simulink model "tqdtqr_rebuild_V3"  (R2021b)
settings: Solver=VariableStepAuto  StartTime=0.0  StopTime=10.0  RelTol=1e-3
undefined symbols (not defined in the file): ATQD_AfterTqMinGain_X_Deg, ATQD_APSCreepBaseTqD_X_kph, ATQD_APSCreepBaseTqD_Y_Deg, ATQD_APSCreepBaseTqR_X_kph, ATQD_APSCreepBaseTqR_Y_Deg, ATQD_APSCreepIterm_X_kph, ATQD_APSCreepIterm_Y_kph, ATQD_APSCreepPterm_X_kph, ATQD_APSCreepPterm_Y_kph, ATQD_APSDecReq_X_kph, ATQD_APSDecReq_Y_mps2, ATQD_APSDecReqCMD_X_kph, ATQD_APSDecReqTs_X_pct, ATQD_APSDecTimeGain_X_Deg, ATQD_APSDecTimeGain_Y_s, ATQD_APSReqLowSpd_X_Deg, ATQD_AutoHoldReleaseBPS_X_Deg, ATQD_AWDLoadTrqnsGain_X_kg, ATQD_AWDLoadTrqnsGain_Y_pct, ATQD_BOSEnBPSPosn_X_kph, ATQD_BOSMap_X_rpm, ATQD_BOSMap_Y_pct, ATQD_CreepBaseTqD_X_kph, ATQD_CreepBaseTqD_Y_Deg, ATQD_CreepBaseTqR_X_kph, ATQD_CreepBaseTqR_Y_Deg, ATQD_CreepBPSDisPosn_X_Deg, ATQD_CreepBPSDisPosnR_X_Deg, ATQD_CreepBPSEnPosn_X_Deg, ATQD_CreepBPSEnPosnR_X_Deg, ATQD_CreepDeltaTq_X_kph, ATQD_CreepIterm_X_kph, ATQD_CreepIterm_Y_kph, ATQD_CreepItermMaxLimit_X_pct, ATQD_CreepPreloadTime_X_kph, ATQD_CreepPreloadTq_X_kph, ATQD_CreepPreloadTq_Y_s, ATQD_CreepProtTq_X_Deg, ATQD_CreepPterm_X_kph, ATQD_CreepPterm_Y_kph, ATQD_CreepRrTqSpRat_X_rpm, ATQD_CreepRrTqSpRat_Y_Nm, ATQD_CreepTargetSpdD_X_pct, ATQD_CreepTargetSpdR_X_pct, ATQD_CreepUpLimitTq_X_rpm, ATQD_DecIneOPDHoldEnDelay_X_Deg, ATQD_DecIneOPDHoldEnDelay_Y_bar, ATQD_ECOTqMapD_X_rpm, ATQD_ECOTqMapD_Y_pct, ATQD_EMTqMapD_X_rpm, ATQD_EMTqMapD_Y_pct, ATQD_EOPDTqMapDCon_X_rpm, ATQD_EOPDTqMapDCon_Y_Deg, ATQD_EstInitVehWeight_X_c, ATQD_FAfterTqCMDGain_X_rpm, ATQD_FAfterTqCMDGain_Y_pct, ATQD_ForceLowSpd_X_Deg, ATQD_ForcePLimitSpd_X_Deg, ATQD_FrLossMAPLowV_X_rpm, ATQD_FrLossMAPLowV_Y_Nm ... (+949)
libraries: simulink x235, hcu_lib x208, tqr x63, tqd x6
(part 16 of 37)

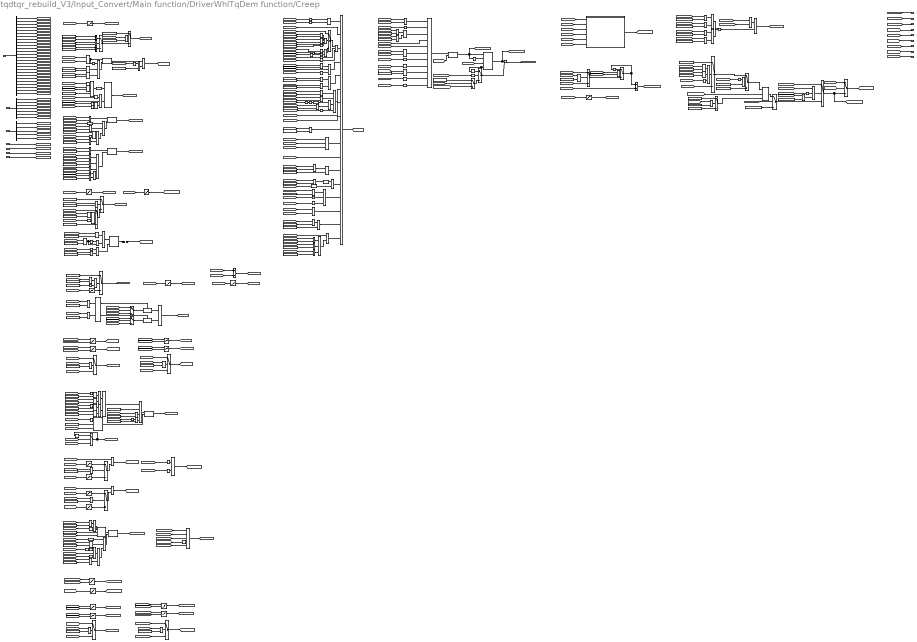
== system tqdtqr_rebuild_V3/Input_Convert/Main function/DriverWhlTqDem function/Creep ==
  note: Calculate creep torque with offset
  note: Creep control reset offset torque
  note: Creep Tq determination
  note: Creep enable parameters
  note: Creep disable parameters
  note: Output final creep torque
  note: Protection condition
  note: Determine brake pedal depth
  note: PI control get torque offset
  note: Preload torque / protect torque
  note: Calculate I value with vehicle speed and error speed
  note: Calculate P value with vehicle speed and error speed
  note: Calculate torque shift R with road slope
  note: Caluclate torque in shift D with road slope
  note: Get error speed from creep speed and vehicle speed
  note: Detemine slope degree
  note: Creep disable judgement
  note: Wheel Status Disable Creep Judgment
  note: Creep enable judgement
  note: calculate creep final speed
  note: Parameters
  note: Creep disable and enable
  note: Creep Tq calculation
  note: Creep offset Tq calculation
  BSCPIn_outputs : Inport
  BSignalConvert_outputs : Inport  Port=2
  BFunction_outputs : Inport  Port=3
  VTQD_PedalMapWhlTq_Nm : Inport  Port=4
  VTQD_LoSpdBrkCtrl_flg : Inport  Port=5
  VTQD_PreLoadPreEn_flg : Inport  Port=6
  VTQD_PedAccTqEn_flg : Inport  Port=7
  AND{,4..7,11..12,15,17,19..26,29} (18 alike) : Logic  AllPortsSameDT=off  OutDataTypeStr=boolean
  AND{1..3,8,13..14,18} (7 alike) : Logic  Inputs=3  AllPortsSameDT=off  OutDataTypeStr=boolean
  AND16 : Logic  Operator=OR  Inputs=3  AllPortsSameDT=off  OutDataTypeStr=boolean
  AND27 : Logic  Inputs=4  AllPortsSameDT=off  OutDataTypeStr=boolean
  Abs : Abs
  Add : Sum  Inputs=+-
  Add1 : Sum
  Add2 : Sum
  Add4 : Sum
  Bus Selector : BusSelector  OutputSignals=VTQD_LowIdleAccPedal_flg,VINP_VehSpeed_kph,VINP_AVHActive_flg,VTQD_ActBPSPosn_pct,VINP_RrRBCActive_flg,VINP_FrEDURealTMTq_Nm,VINP_RrEDURealTMTq_Nm,VINP_FrRBCActive_flg,VVMC_ADASActive_flg,task_time_s,VVMC_APSSpeedCMD_kph,VVMC_APSActive_flg,VVMC_APSReq_enum,VVMC_EstSlope_Deg,VPMM_PowerSta_enum,VINP_EPBSta_enum,VTQD_ActAPSPosn_pct,VVMC_CAASActive_flg,VINP_FrPTCSActive_flg,VINP_RrPTCSActive_flg,VDDM_EPB1Err_flg,VDDM_ESC5Err_flg,VDDM_EPBSigErrCFS_flg,VDDM_VehMalfunLevel_enum,VTQD_LimpHomeAct_flg,VDDM_VCURAPSErrLv2_flg
  Bus Selector1 : BusSelector  OutputSignals=VTQD_RegenMode_enum,VTQD_TMRotateDirction_enum,VTQD_RDCActive_enum,VTQD_BrkSwSta_flg,VTQD_VehActSpd_kph,VTQD_TqTargetShaftSpd_rpm,VTQD_CreepON_flg
  Bus Selector2 : BusSelector  OutputSignals=VTQD_GearActualPosn_enum,VTQD_ActWhlSkipSta_enum,VTQD_APSReq_enum,VTQD_APSReqTimer_s,VTQD_OPDHoldEnRel_flg
  Constant1 : Constant  Value=KTQD_APSCMDEnCreepSpd_kph
  Constant{10..12,21,25,58,62,82} (8 alike) : Constant  Value=ENUM_GEARACTUALPOSN_D
  Constant13 : Constant  Value=KTQD_CreepEnableSpd_kph
  Constant14 : Constant  Value=KTQD_APSCreepLowLimitTq_Nm
  Constant15 : Constant  Value=ZERO_FLOAT
  Constant17 : Constant  Value=ENUM_RDCACTSTA_NOREQUEST
  Constant18 : Constant  Value=ENUM_APSREQ_DECELCTRL  OutDataTypeStr=uint8
  Constant{2,9,20,35..36,38,42..44,49,81} (11 alike) : Constant  Value=ENUM_GEARACTUALPOSN_R
  Constant22 : Constant  Value=KTQD_CreepLowLimitTq_Nm
  Constant23 : Constant  Value=KTQD_CreepPrLoadEnSpd_kph
  Constant24 : Constant  Value=ENUM_RDCACTSTA_NOREQUEST
  Constant26 : Constant  Value=KTQD_CreepDisableSpdofst_kph
  Constant27 : Constant  Value=KTQD_CreepEnableSpdR_kph
  Constant28 : Constant  Value=KTQD_CreepDisableSpdofstR_kph
  Constant29 : Constant  Value=KTQD_CreepEnableSpdR_kph
  Constant{3,87..90} (5 alike) : Constant  Value=KTQD_APSCreepParOvrd_flg
  Constant37 : Constant  Value=ENUM_TMROTATEDIRECTACT_REVERSE  OutDataTypeStr=Inherit: Inherit via back propagation
  Constant39 : Constant  Value=ENUM_TMROTATEDIRECTACT_FORWARD  OutDataTypeStr=Inherit: Inherit via back propagation
  Constant{4,8,52,54,59,64} (6 alike) : Constant  Value=ENUM_REGENLEVEL_OPD
  Constant40 : Constant  Value=KTQD_RBCCreepRecTq_Nm
  Constant41 : Constant  Value=KTQD_RBCCreepRecTq_Nm
  Constant45 : Constant  Value=ENUM_POWERSTA_READY
  Constant46 : Constant  Value=KTQD_CreepEnableSpd_kph
  Constant5 : Constant  Value=ENUM_APSREQ_BRKHOLD  OutDataTypeStr=uint8
  Constant50 : Constant  Value=KTQD_OPDCreepTargetSpdD_kph
  Constant51 : Constant  Value=KTQD_APSReqDisCreep_flg  OutDataTypeStr=uint8
  Constant53 : Constant  Value=KTQD_APSReqDelayTime_s
  Constant55 : Constant  Value=ENUM_EPBSTA_APPLIED  OutDataTypeStr=uint8
  Constant56 : Constant  Value=KTQD_APSReqDisCreep_flg
  Constant6 : Constant  Value=ENUM_GEARACTUALPOSN_P
  Constant60 : Constant  Value=KTQD_OPDCreepDUpLimitTq_Nm
  Constant61 : Constant  Value=KTQD_CreepDisPedTqSpd_kph
  Constant63 : Constant  Value=KTQD_CreepAPSPosn2Launch_pct
  Constant65 : Constant  Value=ENUM_APSREQ_DECELCTRL  OutDataTypeStr=uint8
  Constant66 : Constant  Value=KTQD_TCSCreepDisSpdSW_flg
  Constant67 : Constant  Value=KTQD_TCSCreepDisSpd_kph
  Constant68 : Constant  Value=ENUM_SKIPDISCREEP_LOW
  Constant69 : Constant  Value=KTQD_LowSkipDisCreepDelay_s
  Constant7 : Constant  Value=ENUM_GEARACTUALPOSN_N
  Constant70 : Constant  Value=ENUM_EPBSTA_APPLIED
  Constant71 : Constant  Value=ENUM_SKIPDISCREEP_MEDIUM
  Constant72 : Constant  Value=ENUM_EPBSTA_APPLIED
  Constant73 : Constant  Value=ENUM_SKIPDISCREEP_NORMAL
  Constant74 : Constant  Value=ENUM_SKIPDISCREEP_NORMAL
  Constant75 : Constant  Value=ENUM_SKIPDISCREEP_HIGH
  Constant76 : Constant  Value=ENUM_GEARACTUALPOSN_N
  Constant77 : Constant  Value=ENUM_GEARACTUALPOSN_P
  Constant78 : Constant  Value=ENUM_EPBSTA_APPLIED
  Constant79 : Constant  Value=ENUM_SKIPDISCREEP_NORMAL
  Constant80 : Constant  Value=KTQD_RAPSCreepPreloadSetTime_s
  Constant83 : Constant  Value=KTQD_CreepSlopeLatchSW_flg
  Constant84 : Constant  Value=KTQD_CreepGradeLatchSpd_kph
  Constant85 : Constant  Value=KTQD_CreepLatchGradeDev_Deg
  Constant86 : Constant  Value=KTQD_CreepGradeRecTime_s
  Constant91 : Constant  Value=KTQD_TCSCreepSW_flg
  Constant93 : Constant  Value=KTQD_MALCreepUpLimitTq_Nm
  Constant94 : Constant  Value=ENUM_VEHMALFUNLEVEL_LEVEL3
  Constant97 : Constant  Value=KTQD_FailsafeActiveSW_flg
  Constant98 : Constant  Value=KTQD_FailsafeActiveSW_flg
  Constant99 : Constant  Value=KTQD_FailsafeActiveSW_flg
  Data Type Conversion : DataTypeConversion
  Delay : Delay  DelayLength=1
  Delay1 : Delay  DelayLength=1
  Delay10 : Delay  DelayLength=1  InitialCondition=single(0)
      settings: AttributesFormatString=%<InitialCondition>
  Delay{2..3,6..7} (4 alike) : Delay  DelayLength=1  InitialCondition=boolean(0)
      settings: AttributesFormatString=%<InitialCondition>
  Delay4 : Delay  DelayLength=1  InitialCondition=uint8 (0)
      settings: AttributesFormatString=%<InitialCondition>
  Delay5 : Delay  DelayLength=1  InitialCondition=uint8 (0)
      settings: AttributesFormatString=%<InitialCondition>
  Delay8 : Delay  DelayLength=1  InitialCondition=boolean (0)
      settings: AttributesFormatString=%<InitialCondition>
  Delay9 : Delay  DelayLength=1  InitialCondition=single (0)
      settings: AttributesFormatString=%<InitialCondition>
  DelayEnable : hcu_lib/Basic_Blocks/DelayEnable
  DelayEnable1 : hcu_lib/Basic_Blocks/DelayEnable
  Detect Change : simulink/Logic and Bit Operations/Detect Change  vinit=0  OutDataTypeStr=boolean
  Detect Change1 : simulink/Logic and Bit Operations/Detect Change  vinit=0  OutDataTypeStr=boolean
  Detect Change2 : simulink/Logic and Bit Operations/Detect Change  vinit=0  OutDataTypeStr=boolean
  Detect Increase : simulink/Logic and Bit Operations/Detect Increase  vinit=0  OutDataTypeStr=boolean
  Detect Increase1 : simulink/Logic and Bit Operations/Detect Increase  vinit=0.0  OutDataTypeStr=boolean
  Equal{4,6..8,10..16,19..31,33..54} (46 alike) : RelationalOperator  Operator===  OutDataTypeStr=boolean  RndMeth=Simplest
  Equal17 : RelationalOperator  Operator=<=  OutDataTypeStr=boolean  RndMeth=Simplest
  Equal18 : RelationalOperator  Operator=~=  OutDataTypeStr=boolean  RndMeth=Simplest
  Equal32 : RelationalOperator  OutDataTypeStr=boolean  RndMeth=Simplest
  Equal5 : RelationalOperator  Operator=<=  OutDataTypeStr=boolean  RndMeth=Simplest
  Equal55 : RelationalOperator  OutDataTypeStr=boolean  RndMeth=Simplest
  Equal9 : RelationalOperator  Operator=<=  OutDataTypeStr=boolean  RndMeth=Simplest
  GreaterThan : RelationalOperator  Operator=>  OutDataTypeStr=boolean  RndMeth=Simplest
  GreaterThan1 : RelationalOperator  Operator=>  OutDataTypeStr=boolean  RndMeth=Simplest
  GreaterThan2 : RelationalOperator  OutDataTypeStr=boolean  RndMeth=Simplest
  GreaterThan3 : RelationalOperator  Operator=>  OutDataTypeStr=boolean  RndMeth=Simplest
  GreaterThan4 : RelationalOperator  Operator=<=  OutDataTypeStr=boolean  RndMeth=Simplest
  Ground2 : Ground
  If : If  NumInputs=2  IfExpression=u1 ~= 0  ElseIfExpressions=u2 ~= 0  ShowElse=off
  If Action Subsystem : Subsystem  TreatAsAtomicUnit=on
  If Action Subsystem1 : Subsystem  TreatAsAtomicUnit=on
  Logical Operator{,8..11} (5 alike) : Logic  Operator=NOT  AllPortsSameDT=off  OutDataTypeStr=boolean
  Logical Operator{4,6,15..16,18} (5 alike) : Logic  AllPortsSameDT=off  OutDataTypeStr=boolean
  Logical Operator3 : Logic  Inputs=11  AllPortsSameDT=off  OutDataTypeStr=boolean
  Logical Operator5 : Logic  Operator=OR  AllPortsSameDT=off  OutDataTypeStr=boolean
  Logical Operator7 : Logic  Inputs=3  AllPortsSameDT=off  OutDataTypeStr=boolean
  MTQD_APSCreepBaseTqD_Z_Nm : Lookup_n-D  BreakpointsForDimension1=ATQD_APSCreepBaseTqD_Y_Deg  BreakpointsForDimension2=ATQD_APSCreepBaseTqD_X_kph  Table=MTQD_APSCreepBaseTqD_Z_Nm  ExtrapMethod=Clip  InternalRulePriority=Speed  RndMeth=Simplest  InputSameDT=on
      settings: InputPortMap=u0,u1
  MTQD_APSCreepBaseTqR_Z_Nm : Lookup_n-D  BreakpointsForDimension1=ATQD_APSCreepBaseTqR_Y_Deg  BreakpointsForDimension2=ATQD_APSCreepBaseTqR_X_kph  Table=MTQD_APSCreepBaseTqR_Z_Nm  ExtrapMethod=Clip  InternalRulePriority=Speed  RndMeth=Simplest  InputSameDT=on
      settings: InputPortMap=u0,u1
  MTQD_APSCreepIterm_Z_Nm : Lookup_n-D  BreakpointsForDimension1=ATQD_APSCreepIterm_Y_kph  BreakpointsForDimension2=ATQD_APSCreepIterm_X_kph  Table=MTQD_APSCreepIterm_Z_Nm  ExtrapMethod=Clip  InternalRulePriority=Speed  RndMeth=Simplest  InputSameDT=on
      settings: InputPortMap=u0,u1
  MTQD_APSCreepPterm_Z_Nm : Lookup_n-D  BreakpointsForDimension1=ATQD_APSCreepPterm_Y_kph  BreakpointsForDimension2=ATQD_APSCreepPterm_X_kph  Table=MTQD_APSCreepPterm_Z_Nm  ExtrapMethod=Clip  InternalRulePriority=Speed  RndMeth=Simplest  InputSameDT=on
      settings: InputPortMap=u0,u1
  MTQD_CreepBPSDisPosnR_Y_pct : Lookup_n-D  NumberOfTableDimensions=1  BreakpointsForDimension1=ATQD_CreepBPSDisPosnR_X_Deg  Table=MTQD_CreepBPSDisPosnR_Y_pct  ExtrapMethod=Clip  InternalRulePriority=Speed  RndMeth=Simplest  InputSameDT=on
  MTQD_CreepBPSDisPosn_Y_pct : Lookup_n-D  NumberOfTableDimensions=1  BreakpointsForDimension1=ATQD_CreepBPSDisPosn_X_Deg  Table=MTQD_CreepBPSDisPosn_Y_pct  ExtrapMethod=Clip  InternalRulePriority=Speed  RndMeth=Simplest  InputSameDT=on
  MTQD_CreepBPSEnPosnR_Y_pct : Lookup_n-D  NumberOfTableDimensions=1  BreakpointsForDimension1=ATQD_CreepBPSEnPosnR_X_Deg  Table=MTQD_CreepBPSEnPosnR_Y_pct  ExtrapMethod=Clip  InternalRulePriority=Speed  RndMeth=Simplest  InputSameDT=on
  MTQD_CreepBPSEnPosn_Y_pct : Lookup_n-D  NumberOfTableDimensions=1  BreakpointsForDimension1=ATQD_CreepBPSEnPosn_X_Deg  Table=MTQD_CreepBPSEnPosn_Y_pct  ExtrapMethod=Clip  InternalRulePriority=Speed  RndMeth=Simplest  InputSameDT=on
  MTQD_CreepBaseTqD_Z_Nm : Lookup_n-D  BreakpointsForDimension1=ATQD_CreepBaseTqD_Y_Deg  BreakpointsForDimension2=ATQD_CreepBaseTqD_X_kph  Table=MTQD_CreepBaseTqD_Z_Nm  ExtrapMethod=Clip  InternalRulePriority=Speed  RndMeth=Simplest  InputSameDT=on
      settings: InputPortMap=u0,u1
  MTQD_CreepBaseTqR_Z_Nm : Lookup_n-D  BreakpointsForDimension1=ATQD_CreepBaseTqR_Y_Deg  BreakpointsForDimension2=ATQD_CreepBaseTqR_X_kph  Table=MTQD_CreepBaseTqR_Z_Nm  ExtrapMethod=Clip  InternalRulePriority=Speed  RndMeth=Simplest  InputSameDT=on
      settings: InputPortMap=u0,u1
  MTQD_CreepDeltaTq_Y_Nm : Lookup_n-D  NumberOfTableDimensions=1  BreakpointsForDimension1=ATQD_CreepDeltaTq_X_kph  Table=MTQD_CreepDeltaTq_Y_Nm  ExtrapMethod=Clip  InternalRulePriority=Speed  RndMeth=Simplest  InputSameDT=on
  MTQD_CreepIterm_Z_Nm : Lookup_n-D  BreakpointsForDimension1=ATQD_CreepIterm_Y_kph  BreakpointsForDimension2=ATQD_CreepIterm_X_kph  Table=MTQD_CreepIterm_Z_Nm  ExtrapMethod=Clip  InternalRulePriority=Speed  RndMeth=Simplest  InputSameDT=on
      settings: InputPortMap=u0,u1
  MTQD_CreepPrelaodTq_Z_Nm : Lookup_n-D  BreakpointsForDimension1=ATQD_CreepPreloadTq_Y_s  BreakpointsForDimension2=ATQD_CreepPreloadTq_X_kph  Table=MTQD_CreepPreloadTq_Z_Nm  ExtrapMethod=Clip  InternalRulePriority=Speed  RndMeth=Simplest  InputSameDT=on
      settings: InputPortMap=u0,u1
  MTQD_CreepPreloadTime_Y_s : Lookup_n-D  NumberOfTableDimensions=1  BreakpointsForDimension1=ATQD_CreepPreloadTime_X_kph  Table=MTQD_CreepPreloadTime_Y_s  ExtrapMethod=Clip  InternalRulePriority=Speed  RndMeth=Simplest  InputSameDT=on
  MTQD_CreepProtTq_Y_Nm : Lookup_n-D  NumberOfTableDimensions=1  BreakpointsForDimension1=ATQD_CreepProtTq_X_Deg  Table=MTQD_CreepProtTq_Y_Nm  ExtrapMethod=Clip  InternalRulePriority=Speed  RndMeth=Simplest  InputSameDT=on
  MTQD_CreepPterm_Z_Nm : Lookup_n-D  BreakpointsForDimension1=ATQD_CreepPterm_Y_kph  BreakpointsForDimension2=ATQD_CreepPterm_X_kph  Table=MTQD_CreepPterm_Z_Nm  ExtrapMethod=Clip  InternalRulePriority=Speed  RndMeth=Simplest  InputSameDT=on
      settings: InputPortMap=u0,u1
  "MTQD_CreepTargetSpdD_Y_kph " : Lookup_n-D  NumberOfTableDimensions=1  BreakpointsForDimension1=ATQD_CreepTargetSpdD_X_pct  Table=MTQD_CreepTargetSpdD_Y_kph  ExtrapMethod=Clip  InternalRulePriority=Speed  RndMeth=Simplest  InputSameDT=on
  MTQD_CreepTargetSpdR_Y_kph : Lookup_n-D  NumberOfTableDimensions=1  BreakpointsForDimension1=ATQD_CreepTargetSpdR_X_pct  Table=MTQD_CreepTargetSpdR_Y_kph  ExtrapMethod=Clip  InternalRulePriority=Speed  RndMeth=Simplest  InputSameDT=on
  MTQD_CreepUpLimitTq_Y_Nm : Lookup_n-D  NumberOfTableDimensions=1  BreakpointsForDimension1=ATQD_CreepUpLimitTq_X_rpm  Table=MTQD_CreepUpLimitTq_Y_Nm  ExtrapMethod=Clip  InternalRulePriority=Speed  RndMeth=Simplest  InputSameDT=on
  MTQD_OPDHoldEnSpd_Y_kph : Lookup_n-D  NumberOfTableDimensions=1  BreakpointsForDimension1=ATQD_OPDHoldEnSpd_X_Deg  Table=MTQD_OPDHoldEnSpd_Y_kph  InternalRulePriority=Speed  RndMeth=Simplest  InputSameDT=on
  MTQD_WhlSkipDisCreep_Y_enum : Lookup_n-D  NumberOfTableDimensions=1  BreakpointsForDimension1=ATQD_WhlSkipDisCreep_X_enum  BreakpointsForDimension1DataTypeStr=uint8  Table=MTQD_WhlSkipDisCreep_Y_enum  TableDataTypeStr=uint8  IntermediateResultsDataTypeStr=uint8  ExtrapMethod=Clip  UseLastTableValue=on  InternalRulePriority=Speed  OutDataTypeStr=uint8  RndMeth=Simplest  InputSameDT=on
  Merge : Merge
  NOT{,1..26} (27 alike) : Logic  Operator=NOT  AllPortsSameDT=off  OutDataTypeStr=boolean
  OR{,2..3,6..11,17..22,25} (16 alike) : Logic  Operator=OR  AllPortsSameDT=off  OutDataTypeStr=boolean
  OR1 : Logic  Operator=OR  Inputs=17  AllPortsSameDT=off  OutDataTypeStr=boolean
  OR{5,12..15} (5 alike) : Logic  Operator=OR  Inputs=3  AllPortsSameDT=off  OutDataTypeStr=boolean
  OR16 : Logic  Operator=OR  Inputs=4  AllPortsSameDT=off  OutDataTypeStr=boolean
  OR23 : Logic  AllPortsSameDT=off  OutDataTypeStr=boolean
  OR24 : Logic  Operator=OR  Inputs=5  AllPortsSameDT=off  OutDataTypeStr=boolean
  OR4 : Logic  Inputs=4  AllPortsSameDT=off  OutDataTypeStr=boolean
  Relational Operator : RelationalOperator  OutDataTypeStr=boolean  RndMeth=Simplest
  Relational Operator1 : RelationalOperator  Operator=<  OutDataTypeStr=boolean  RndMeth=Simplest
  Relational Operator2 : RelationalOperator  Operator=>  OutDataTypeStr=boolean  RndMeth=Simplest
  Relational Operator3 : RelationalOperator  Operator=>  OutDataTypeStr=boolean  RndMeth=Simplest
  Relational Operator4 : RelationalOperator  Operator=>  OutDataTypeStr=boolean  RndMeth=Simplest
  Relational Operator5 : RelationalOperator  Operator=<=  OutDataTypeStr=boolean  RndMeth=Simplest
  Relational Operator6 : RelationalOperator  Operator=<=  OutDataTypeStr=boolean  RndMeth=Simplest
  Relational Operator7 : RelationalOperator  Operator=<=  OutDataTypeStr=boolean  RndMeth=Simplest
  Relay : Relay  OnSwitchValue=KTQD_OPDCreepEnGrade_Deg  OffSwitchValue=KTQD_OPDCreepDisGrade_Deg  OnOutputValue=TRUE  OffOutputValue=FALSE  OutDataTypeStr=boolean
      settings: AttributesFormatString=|
      | ON:%<OnSwitchValue>
      | OFF:%<OffSwitchValue>
  SR_Latch{,1..7} (8 alike) : hcu_lib/Basic_Blocks/SR_Latch
  Saturation Dynamic : simulink/Discontinuities/Saturation Dynamic  OutMin=[]  OutMax=[]  OutDataTypeStr=Inherit: Same as second input  OutDataType=fixdt(1, 16)  OutScaling=2^-10  DoSatur=off
  Switch{,1..22,24..25} (25 alike) : Switch  Criteria=u2 ~= 0
      Switch settings: AttributesFormatString=%<Criteria>
      Switch1 settings: AttributesFormatString=%<Criteria>
      Switch10 settings: AttributesFormatString=%<Criteria>
      Switch11 settings: AttributesFormatString=%<Criteria>
      Switch12 settings: AttributesFormatString=%<Criteria>
      Switch13 settings: AttributesFormatString=%<Criteria>
      Switch14 settings: AttributesFormatString=%<Criteria>
      Switch15 settings: AttributesFormatString=%<Criteria>
      Switch16 settings: AttributesFormatString=%<Criteria>
      Switch17 settings: AttributesFormatString=%<Criteria>
      Switch18 settings: AttributesFormatString=%<Criteria>
      Switch19 settings: AttributesFormatString=%<Criteria>
      Switch2 settings: AttributesFormatString=%<Criteria>
      Switch20 settings: AttributesFormatString=%<Criteria>
      Switch21 settings: AttributesFormatString=%<Criteria>
      Switch22 settings: AttributesFormatString=%<Criteria>
      Switch25 settings: AttributesFormatString=%<Criteria>
      Switch4 settings: AttributesFormatString=%<Criteria>
      Switch5 settings: AttributesFormatString=%<Criteria>
      Switch6 settings: AttributesFormatString=%<Criteria>
      Switch8 settings: AttributesFormatString=%<Criteria>
      Switch9 settings: AttributesFormatString=%<Criteria>
  Switch Case Action Subsystem : Subsystem  TreatAsAtomicUnit=on
  Terminator3 : Terminator
  Timer : hcu_lib/Basic_Blocks/Timer
  Unit Delay : UnitDelay  InitialCondition=single(0)  SampleTime=-1  HasFrameUpgradeWarning=on
      settings: AttributesFormatString=%<InitialCondition>
  Unit Delay1 : UnitDelay  InitialCondition=boolean(0)  SampleTime=-1  HasFrameUpgradeWarning=on
      settings: AttributesFormatString=%<InitialCondition>
  VTQD_CreepEnable_flg : Outport
  VTQD_CreepWhlTqDem_Nm : Outport  Port=2
  VTQD_CreepPrLoadEnable_flg : Outport  Port=3
  VTQD_OPDOn2Off_flg : Outport  Port=4
  VTQD_CreepProtTqEn_flg : Outport  Port=5
  VTQD_CreepBaseTqD_Nm : Outport  Port=6
  VTQD_CreepBaseTqR_Nm : Outport  Port=7
  VTQD_HighBPSPosn_flg : Outport  Port=8
  VTQD_CreepTCSActive_flg : Outport  Port=9
  wires:
  [VTQD_CreepTotalOfstTq_Nm] -> Add2/2
  If Action Subsystem1/1(VTQD_CreepTotalOfstTq_Nm) -> [VTQD_CreepTotalOfstTq_Nm]
  [VTQD_ActBPSPosn_pct] -> If Action Subsystem1/5(VTQD_ActBPSPosn_pct)
  [VTQD_CreepDeltaTq_Nm] -> If Action Subsystem1/4(VTQD_CreepDeltaTq_Nm)
  [VTQD_CreepItermInp_c] -> If Action Subsystem1/3(VTQD_CreepItermInp_c)
  [VTQD_CreepPtermInp_c] -> If Action Subsystem1/2(VTQD_CreepPtermInp_c)
  AND6/1 -> [VTQD_ActBPSPosnInRange_flg]  "VTQD_ActBPSPosnInRange_flg"
  NOT4/1 -> Logical Operator3/2
  [VTQD_OPDOn2Off_flg] -> NOT4/1
  NOT3/1 -> Logical Operator3/8
  NOT/1 -> Logical Operator3/7
  Merge/1 -> [VTQD_CreepFinalSpd_kph]  "VTQD_CreepFinalSpd_kph"
  Switch Case Action Subsystem/1(Out1) -> Merge/2
  If Action Subsystem/1(Out1) -> Merge/1
  If/2 -> Switch Case Action Subsystem/Action
  If/1 -> If Action Subsystem/Action
  Equal12/1 -> If/2
  Constant2/1 -> Equal12/2
  [VTQD_GearActualPosn_enum] -> Equal12/1
  Equal13/1 -> If/1
  Constant12/1 -> Equal13/2
  [VTQD_GearActualPosn_enum] -> Equal13/1
  [VTQD_HighBPSPosn_flg] -> OR1/2
  [VVMC_ADASActive_flg] -> NOT3/1
  [VTQD_RBCActive_flg] -> NOT/1
  [VTQD_CreepEnSpd_kph] -> Equal9/2
  OR1/1 -> [VTQD_CreepDisable_flg]  "VTQD_CreepDisable_flg"
  [VTQD_CreepDisable_flg] -> SR_Latch/2
  [VTQD_RegenMode_enum] -> Equal11/1
  Constant8/1 -> Equal11/2
  [VTQD_CreepON_flg] -> NOT2/1
  Equal10/1 -> OR/2
  Equal6/1 -> OR/1
  Constant7/1 -> Equal10/2
  [VTQD_GearActualPosn_enum] -> Equal10/1
  Constant6/1 -> Equal6/2
  [VTQD_GearActualPosn_enum] -> Equal6/1
  [VTQD_LowIdleAccPedal_flg] -> NOT1/1
  [VTQD_LowIdleAccPedal_flg] -> AND2/2
  GreaterThan1/1 -> AND2/1
  [VTQD_CreepDisSpd_kph] -> GreaterThan1/2
  [VTQD_VehActSpd_kph] -> GreaterThan1/1
  Unit Delay/1 -> GreaterThan/2
  [VTQD_CreepWhlTqDem_Nm] -> Unit Delay/1
  [VTQD_PedalMapWhlTq_Nm] -> GreaterThan/1
  VTQD_PedalMapWhlTq_Nm/1 -> [VTQD_PedalMapWhlTq_Nm]
  [VTQD_LowBPSPosn_flg] -> Logical Operator3/4
  Equal7/1 -> Logical Operator5/1
  [VTQD_GearActualPosn_enum] -> Equal8/1
  Equal8/1 -> Logical Operator5/2
  Constant20/1 -> Equal7/2
  Constant21/1 -> Equal8/2
  [VTQD_GearActualPosn_enum] -> Equal7/1
  [VTQD_LowIdleAccPedal_flg] -> Logical Operator3/5
  [VTQD_VehActSpd_kph] -> Equal9/1
  Logical Operator5/1 -> Logical Operator3/3
  Equal9/1 -> Logical Operator3/6
  Logical Operator3/1 -> SR_Latch/1
  SR_Latch3/1 -> Terminator3/1
  Equal14/1 -> Logical Operator3/9
  Switch/1 -> Switch4/3
  [VTQD_CreepEnable_flg] -> Switch/2
  Constant15/1 -> Switch/3
  [VTQD_LoSpdBrkCtrl_flg] -> NOT9/1
  NOT9/1 -> Logical Operator3/10
  VTQD_LoSpdBrkCtrl_flg/1 -> [VTQD_LoSpdBrkCtrl_flg]
  Switch1/1 -> If Action Subsystem/1(In1)
  [VTQD_CreepTargetSpdD_kph] -> Switch1/3
  [VVMC_APSActive_flg] -> Switch1/2
  [VVMC_APSActive_flg] -> Switch2/2
  Switch2/1 -> Switch Case Action Subsystem/1(In1)
  [VVMC_APSActive_flg] -> OR3/1
  [VTQD_CreepON_flg] -> OR3/2
  OR3/1 -> Logical Operator3/1
  NOT2/1 -> AND/2
  AND/1 -> OR1/1
  [VVMC_APSActive_flg] -> NOT5/1
  NOT5/1 -> AND/1
  [VTQD_CreepBaseTqDInp_Nm] -> Switch3/3
  [VTQD_CreepBaseTqRInp_Nm] -> Switch3/1
  Constant9/1 -> Equal16/2
  [VTQD_GearActualPosn_enum] -> Equal16/1
  Equal16/1 -> Switch3/2
  Timer/1 -> [VTQD_CreepPreloadTime_s], Relational Operator/1  "VTQD_CreepPreloadTime_s"
  [task_time_s] -> Timer/3
  Relational Operator/1 -> [VTQD_CreepEnable_flg]  "VTQD_CreepEnable_flg"
  SR_Latch/1 -> [VTQD_CreepPrLoadEnable_flg], NOT8/1, Timer/1  "VTQD_CreepPrLoadEnable_flg"
  NOT8/1 -> Timer/2
  [VTQD_CreepEnable_flg] -> NOT10/1
  NOT10/1 -> AND3/2
  [VTQD_CreepPreloadTq_Nm] -> Switch4/1
  [VTQD_CreepPrLoadEnable_flg] -> AND3/1
  AND3/1 -> Switch4/2
  [VINP_VehSpeed_kph] -> Equal17/1
  Constant23/1 -> Equal17/2
  Equal17/1 -> AND3/3
  AND1/1 -> OR1/3
  AND2/1 -> OR1/4
  OR/1 -> OR1/5
  [VVMC_ADASActive_flg] -> OR1/8
  [VTQD_RDCActive_enum] -> Equal14/1
  Constant17/1 -> Equal14/2
  Constant24/1 -> Equal18/2
  [VTQD_RDCActive_enum] -> Equal18/1
  Equal18/1 -> OR1/9
  [VINP_AVHActive_flg] -> OR1/11
  [VTQD_GearActualPosn_enum] -> Equal19/1
  Constant25/1 -> Equal19/2
  Constant35/1 -> Equal21/2
  Add1/1 -> Switch5/1
  [VTQD_GearActualPosn_enum] -> Equal21/1
  Equal21/1 -> Switch5/2
  Constant27/1 -> Add1/1
  Add4/1 -> Switch5/3
  Constant13/1 -> Add4/1
  Constant26/1 -> Add4/2
  Constant28/1 -> Add1/2
  [VVMC_APSSpeedCMD_kph] -> Relational Operator1/1
  [VVMC_APSActive_flg] -> AND5/1
  Constant1/1 -> Relational Operator1/2
  Equal20/1 -> OR5/2
  OR5/1 -> AND5/2
  Constant5/1 -> Equal20/2
  [VVMC_APSReq_enum] -> Equal20/1
  Relational Operator1/1 -> OR5/1
  AND7/1 -> [VTQD_CreepProtTqEn_flg]  "VTQD_CreepProtTqEn_flg"
  Equal25/1 -> Logical Operator6/1
  [VTQD_GearActualPosn_enum] -> Equal25/1
  [VTQD_CreepProtTq_Nm] -> Relational Operator2/1
  Constant38/1 -> Equal25/2
  Relational Operator2/1 -> AND7/1
  [VTQD_CreepActWhlTqDem_Nm] -> Relational Operator2/2
  [VTQD_TMRotateDirction_enum] -> Equal26/1
  Constant39/1 -> Equal26/2
  Logical Operator4/1 -> OR6/1
  [VTQD_GearActualPosn_enum] -> Equal23/1
  [VTQD_TMRotateDirction_enum] -> Equal24/1
  Constant11/1 -> Equal23/2
  Equal23/1 -> Logical Operator4/1
  Equal24/1 -> Logical Operator4/2
  Constant37/1 -> Equal24/2
  OR6/1 -> AND7/2
  Equal26/1 -> Logical Operator6/2
  Logical Operator6/1 -> OR6/2
  Switch4/1 -> [VTQD_CreepActWhlTqDem_Nm], Switch7/3  "VTQD_CreepActWhlTqDem_Nm"
  [VTQD_CreepProtTqEn_flg] -> Switch7/2
  Switch7/1 -> [VTQD_CreepWhlTqDem_Nm]  "VTQD_CreepWhlTqDem_Nm"
  [VTQD_CreepProtTq_Nm] -> Switch7/1
  Relational Operator4/1 -> AND8/2
  NOT7/1 -> AND8/1
  OR23/1 -> [VTQD_RBCActive_flg]  "VTQD_RBCActive_flg"
  AND8/1 -> SR_Latch1/2  "VTQD_RBCActiveRec_flg"
  Constant41/1 -> Relational Operator4/2
  OR7/1 -> NOT7/1, SR_Latch1/1
  [VINP_FrEDURealTMTq_Nm] -> Relational Operator4/1
  Constant40/1 -> Relational Operator3/2
  [VINP_RrEDURealTMTq_Nm] -> Relational Operator3/1
  Relational Operator3/1 -> AND8/3
  [VINP_RrRBCActive_flg] -> OR7/1
  [VINP_FrRBCActive_flg] -> OR7/2
  [VVMC_EstSlope_Deg] -> Relay/1
  Ground2/1 -> [VTQD_OPDOn2Off_flg]  "VTQD_OPDOn2Off_flg"
  [VPMM_PwrSta_enum] -> Equal30/1
  Equal29/1 -> OR2/2
  [VTQD_GearActualPosn_enum] -> Equal29/1
  Equal4/1 -> GreaterThan3/2, Unit Delay1/1
  Constant4/1 -> Equal4/2
  [VTQD_LowIdleAccPedal_flg] -> NOT6/1
  GreaterThan3/1 -> AND4/2
  Equal30/1 -> AND4/1
  Constant45/1 -> Equal30/2
  Constant44/1 -> Equal29/2
  NOT6/1 -> OR2/1
  [VTQD_RegenMode_enum] -> Equal4/1
  OR2/1 -> SR_Latch3/2
  Unit Delay1/1 -> GreaterThan3/1
  AND4/1 -> SR_Latch3/1
  Constant43/1 -> Equal28/2
  [VVMC_EstSlope_Deg] -> MTQD_CreepBPSDisPosnR_Y_pct/1
  Equal27/1 -> Switch8/2
  MTQD_CreepBPSDisPosn_Y_pct/1 -> Switch9/3  "VTQD_CreepBPSDisPosn_pct"
  [VTQD_ActBPSPosn_pct] -> GreaterThan2/1
  GreaterThan2/1 -> [VTQD_HighBPSPosn_flg]  "VTQD_HighBPSPosn_flg"
  Switch9/1 -> GreaterThan2/2
  Equal5/1 -> [VTQD_LowBPSPosn_flg]  "VTQD_LowBPSPosn_flg"
  Equal28/1 -> Switch9/2
  [VVMC_EstSlope_Deg] -> MTQD_CreepBPSDisPosn_Y_pct/1
  [VTQD_GearActualPosn_enum] -> Equal28/1
  Constant42/1 -> Equal27/2
  Switch8/1 -> Equal5/2
  [VVMC_EstSlope_Deg] -> MTQD_CreepBPSEnPosnR_Y_pct/1
  MTQD_CreepBPSEnPosn_Y_pct/1 -> Switch8/3  "VTQD_CreepBPSEnPosn_pct"
  MTQD_CreepBPSDisPosnR_Y_pct/1 -> Switch9/1  "VTQD_CreepBPSDisPosnR_pct"
  [VTQD_GearActualPosn_enum] -> Equal27/1
  MTQD_CreepBPSEnPosnR_Y_pct/1 -> Switch8/1  "VTQD_CreepBPSEnPosnR_pct"
  [VTQD_ActBPSPosn_pct] -> Equal5/1
  [VVMC_EstSlope_Deg] -> MTQD_CreepBPSEnPosn_Y_pct/1
  NOT11/1 -> Logical Operator3/11
  [VTQD_PreLoadPreEn_flg] -> NOT11/1
  [VTQD_VehActSpd_kph] -> MTQD_CreepPreloadTime_Y_s/1
  Delay/1 -> Switch10/1
  [VTQD_CreepEnable_flg] -> Delay1/1
  Delay1/1 -> Switch10/2
  Switch10/1 -> Delay/1, Timer/4, Relational Operator/2
  MTQD_CreepPterm_Z_Nm/1 -> [VTQD_CreepPterm_c]  "VTQD_CreepPterm_c"
  Add/1 -> [VTQD_CreepErrSpd_kph]  "VTQD_CreepErrSpd_kph"
  [VINP_VehSpeed_kph] -> MTQD_CreepPrelaodTq_Z_Nm/2
  [VTQD_CreepCtrlGrade_Deg] -> MTQD_CreepBaseTqR_Z_Nm/1
  MTQD_CreepBaseTqD_Z_Nm/1 -> [VTQD_CreepBaseTqD_Nm]  "VTQD_CreepBaseTqD_Nm"
  [VTQD_VehActSpd_kph] -> MTQD_CreepBaseTqD_Z_Nm/2
  MTQD_CreepDeltaTq_Y_Nm/1 -> [VTQD_CreepDeltaTq_Nm]  "VTQD_CreepDeltaTq_Nm"
  [VTQD_VehActSpd_kph] -> Add/2
  [VTQD_VehActSpd_kph] -> MTQD_CreepBaseTqR_Z_Nm/2
  [VTQD_CreepPreloadTime_s] -> MTQD_CreepPrelaodTq_Z_Nm/1
  MTQD_CreepBaseTqR_Z_Nm/1 -> [VTQD_CreepBaseTqR_Nm]  "VTQD_CreepBaseTqR_Nm"
  [VTQD_CreepFinalSpd_kph] -> Add/1
  [VTQD_CreepCtrlGrade_Deg] -> MTQD_CreepBaseTqD_Z_Nm/1
  MTQD_CreepPrelaodTq_Z_Nm/1 -> [VTQD_CreepPreloadTq_Nm]  "VTQD_CreepPreloadTq_Nm"
  MTQD_CreepProtTq_Y_Nm/1 -> [VTQD_CreepProtTq_Nm]  "VTQD_CreepProtTq_Nm"
  [VTQD_CreepErrSpd_kph] -> MTQD_CreepDeltaTq_Y_Nm/1
  [VVMC_EstSlope_Deg] -> MTQD_CreepProtTq_Y_Nm/1
  [VTQD_GearActualPosn_enum] -> Detect Change/1
  [VVMC_EstSlope_Deg] -> MTQD_OPDHoldEnSpd_Y_kph/1
  MTQD_OPDHoldEnSpd_Y_kph/1 -> [VTQD_OPDHoldEnSpd_kph]  "VTQD_OPDHoldEnSpd_kph"
  [VTQD_LowBPSPosn_flg] -> NOT12/1
  [VTQD_HighBPSPosn_flg] -> NOT13/1
  NOT12/1 -> AND6/1
  NOT13/1 -> AND6/2
  [VTQD_RBCActive_flg] -> OR1/7
  Constant53/1 -> Equal32/2
  [VTQD_APSReqTimer_s] -> Equal32/1
  Equal32/1 -> OR8/2
  Data Type Conversion/1 -> OR8/1  "VTQD_OPDCreepGrade_flg"
  [VTQD_APSReq_enum] -> Equal15/1
  Constant18/1 -> Equal15/2
  Equal15/1 -> AND11/1
  Constant51/1 -> AND11/2
  AND11/1 -> OR1/12
  Constant55/1 -> Equal34/2
  [VINP_EPBSta_enum] -> Equal34/1
  Equal31/1 -> AND12/1
  AND12/1 -> Switch12/2
  Switch12/1 -> [VTQD_CreepTargetSpdD_kph]  "VTQD_CreepTargetSpdD_kph"
  Constant56/1 -> NOT14/1
  NOT14/1 -> AND12/2
  [VTQD_RegenMode_enum] -> Equal31/1
  Constant52/1 -> Equal31/2
  Constant50/1 -> Switch12/1
  Saturation Dynamic/1 -> Switch/1
  [VTQD_VehActSpd_kph] -> GreaterThan4/1
  Constant61/1 -> GreaterThan4/2
  NOT1/1 -> AND1/2
  Switch15/1 -> AND1/1
  [VTQD_OPDHoldEnRel_flg] -> Switch15/1
  [VTQD_GearActualPosn_enum] -> Equal37/1
  Constant62/1 -> Equal37/2
  AND14/1 -> Switch15/2
  GreaterThan4/1 -> AND14/2
  Equal37/1 -> AND14/1
  [VVMC_APSSpeedCMD_kph] -> Switch1/1
  [VVMC_APSSpeedCMD_kph] -> Switch2/1
  GreaterThan/1 -> AND15/2
  AND15/1 -> Switch15/3
  NOT15/1 -> AND15/1
  [VVMC_APSActive_flg] -> NOT15/1
  [VTQD_ActAPSPosn_pct] -> Relational Operator5/1
  Constant63/1 -> Relational Operator5/2
  Relational Operator5/1 -> AND14/3
  [VTQD_RegenMode_enum] -> Equal38/1
  Constant64/1 -> Equal38/2
  Detect Change/1 -> OR9/2
  OR9/1 -> OR1/13
  Equal38/1 -> Detect Increase/1
  Detect Increase/1 -> OR9/1
  [VTQD_VehActSpd_kph] -> MTQD_CreepIterm_Z_Nm/1
  MTQD_CreepIterm_Z_Nm/1 -> [VTQD_CreepIterm_c]  "VTQD_CreepIterm_c"
  [VTQD_CreepErrSpd_kph] -> MTQD_CreepIterm_Z_Nm/2
  [VVMC_APSReq_enum] -> Equal39/1
  Constant65/1 -> Equal39/2
  Equal39/1 -> OR5/3
  [VTQD_VehActSpd_kph] -> MTQD_CreepPterm_Z_Nm/1
  [VTQD_CreepErrSpd_kph] -> MTQD_CreepPterm_Z_Nm/2
  [VTQD_LoSpdBrkCtrl_flg] -> AND16/1
  AND16/1 -> OR1/10
  [VVMC_CAASActive_flg] -> OR10/1
  [VTQD_PedAccTqEn_flg] -> OR10/2
  OR10/1 -> OR1/15
  Constant54/1 -> Equal33/2
  Equal22/1 -> Switch6/2
  [VTQD_GearActualPosn_enum] -> Equal22/1
  Equal33/1 -> AND17/1
  [VVMC_APSActive_flg] -> NOT16/1
  NOT16/1 -> AND17/2
  Constant46/1 -> Switch13/3
  [VTQD_RegenMode_enum] -> Equal33/1
  [VTQD_OPDHoldEnSpd_kph] -> Switch13/1
  Switch6/1 -> [VTQD_CreepEnSpd_kph]  "VTQD_CreepEnSpd_kph"
  Switch13/1 -> Switch6/3
  Constant29/1 -> Switch6/1
  Constant36/1 -> Equal22/2
  AND17/1 -> Switch13/2
  [VVMC_APSActive_flg] -> NOT17/1
  NOT17/1 -> OR4/4
  OR8/1 -> OR4/3
  Equal19/1 -> OR4/2
  Equal11/1 -> OR4/1
  OR4/1 -> OR1/6
  [VVMC_APSActive_flg] -> NOT18/1
  NOT18/1 -> AND13/3
  AND13/1 -> Switch14/2
  [VTQD_RegenMode_enum] -> Equal36/1
  Equal35/1 -> AND13/1
  Constant58/1 -> Equal35/2
  [VTQD_GearActualPosn_enum] -> Equal35/1
  Constant59/1 -> Equal36/2
  Equal36/1 -> AND13/2
  Constant60/1 -> Switch14/1
  [VINP_RrPTCSActive_flg] -> NOT20/1
  SR_Latch4/1 -> [VTQD_CreepTCSActive_flg]  "VTQD_CreepTCSActive_flg"
  [VINP_FrPTCSActive_flg] -> NOT19/1
  NOT20/1 -> AND19/2
  OR12/1 -> SR_Latch4/2
  OR11/1 -> AND18/2
  Detect Increase1/1 -> SR_Latch4/1
  [VTQD_CreepEnable_flg] -> Delay6/1
  Delay6/1 -> AND18/1
  Delay7/1 -> OR12/1
  Constant91/1 -> AND18/3
  AND18/1 -> Detect Increase1/1
  [VTQD_CreepDisable_flg] -> Delay7/1
  [VINP_FrPTCSActive_flg] -> OR11/1
  [VINP_RrPTCSActive_flg] -> OR11/2
  NOT19/1 -> AND19/1
  [VTQD_CreepTCSActive_flg] -> NOT21/1
  NOT21/1 -> AND1/3
  NOT22/1 -> AND2/3
  [VTQD_CreepTCSActive_flg] -> NOT22/1
  AND19/1 -> OR12/3
  [VTQD_BrkSwSta_flg] -> OR12/2
  Switch5/1 -> Switch16/3
  Switch16/1 -> [VTQD_CreepDisSpd_kph]  "VTQD_CreepDisSpd_kph"
  AND20/1 -> Switch16/2
  [VTQD_CreepTCSActive_flg] -> AND20/1
  Constant66/1 -> AND20/2
  Constant67/1 -> Switch16/1
  [VTQD_ActWhlSkipSta_enum] -> MTQD_WhlSkipDisCreep_Y_enum/1
  Delay2/1 -> AND21/2
  AND21/1 -> DelayEnable/1
  Constant69/1 -> DelayEnable/2
  Equal40/1 -> AND21/1
  [VTQD_CreepEnable_flg] -> Delay3/1
  MTQD_WhlSkipDisCreep_Y_enum/1 -> [VTQD_WhlSkipDisCreep_enum]  "VTQD_WhlSkipDisCreep_enum"
  [VTQD_CreepEnable_flg] -> Delay2/1
  [VTQD_WhlSkipDisCreep_enum] -> Equal40/1
  DelayEnable/1 -> SR_Latch2/1
  [task_time_s] -> DelayEnable/3
  Constant68/1 -> Equal40/2
  [VTQD_LowIdleAccPedal_flg] -> NOT23/1
  [VTQD_GearActualPosn_enum] -> Detect Change1/1
  [VINP_EPBSta_enum] -> Equal41/1
  Constant70/1 -> Equal41/2
  OR13/1 -> SR_Latch2/2  "VTQD_LowSkipDisRset_flg"
  Constant71/1 -> Equal42/2
  [VTQD_WhlSkipDisCreep_enum] -> Equal42/1
  SR_Latch2/1 -> [VTQD_LowSkipDisCreep_flg]  "VTQD_LowSkipDisCreep_flg"
  Constant72/1 -> Equal43/2
  [VINP_EPBSta_enum] -> Equal43/1
  [VTQD_GearActualPosn_enum] -> Detect Change2/1
  [VTQD_LowIdleAccPedal_flg] -> NOT24/1
  SR_Latch5/1 -> [VTQD_MediumSkipDisCreep_flg]  "VTQD_MediumSkipDisCreep_flg"
  OR14/1 -> SR_Latch5/2  "VTQD_MediumSkipDisRset_flg"
  Equal42/1 -> SR_Latch5/1
  Constant75/1 -> Equal45/2
  [VTQD_WhlSkipDisCreep_enum] -> Equal45/1
  Equal45/1 -> SR_Latch6/1
  [VTQD_GearActualPosn_enum] -> Equal46/1
  Constant76/1 -> Equal46/2
  Constant77/1 -> Equal47/2
  [VTQD_GearActualPosn_enum] -> Equal47/1
  [VINP_EPBSta_enum] -> Equal48/1
  Constant78/1 -> Equal48/2
  OR16/1 -> SR_Latch6/2  "VTQD_HighSkipDisRset_flg"
  SR_Latch6/1 -> [VTQD_HighSkipDisCreep_flg]  "VTQD_HighSkipDisCreep_flg"
  [VTQD_BrkSwSta_flg] -> OR15/2
  NOT23/1 -> OR15/3
  OR15/1 -> AND22/1
  Constant73/1 -> Equal44/2
  [VTQD_WhlSkipDisCreep_enum] -> Equal44/1
  Equal44/1 -> AND22/2
  Detect Change1/1 -> OR13/1
  Equal41/1 -> OR13/2
  AND22/1 -> OR13/3
  [VTQD_BrkSwSta_flg] -> OR17/1
  NOT24/1 -> OR17/2
  OR17/1 -> AND23/1
  Constant74/1 -> Equal49/2
  [VTQD_WhlSkipDisCreep_enum] -> Equal49/1
  Equal49/1 -> AND23/2
  Detect Change2/1 -> OR14/1
  Equal43/1 -> OR14/2
  AND23/1 -> OR14/3
  [VTQD_HighBPSPosn_flg] -> AND24/1
  [VTQD_WhlSkipDisCreep_enum] -> Equal50/1
  Constant79/1 -> Equal50/2
  Equal50/1 -> AND24/2
  Equal46/1 -> OR16/1
  Equal47/1 -> OR16/2
  Equal48/1 -> OR16/3
  AND24/1 -> OR16/4
  Delay3/1 -> NOT25/1
  NOT25/1 -> OR15/1
  Logical Operator8/1 -> Logical Operator7/2
  [VDDM_EPBSigErrCFS_flg] -> Logical Operator11/1
  Logical Operator11/1 -> Logical Operator7/3
  Equal34/1 -> Logical Operator7/1
  Logical Operator7/1 -> OR1/14
  [VTQD_MediumSkipDisCreep_flg] -> AND16/2
  [VTQD_HighSkipDisCreep_flg] -> AND16/3
  Switch17/1 -> Switch10/3
  [VVMC_APSActive_flg] -> Switch17/2
  Constant80/1 -> Switch17/1
  [VTQD_ActBPSPosn_pct] -> "MTQD_CreepTargetSpdD_Y_kph "/1
  "MTQD_CreepTargetSpdD_Y_kph "/1 -> Switch12/3
  [VTQD_ActBPSPosn_pct] -> MTQD_CreepTargetSpdR_Y_kph/1
  MTQD_CreepTargetSpdR_Y_kph/1 -> [VTQD_CreepTargetSpdR_kph]  "VTQD_CreepTargetSpdR_kph"
  [VTQD_CreepTargetSpdR_kph] -> Switch2/3
  Constant10/1 -> Equal51/2
  AND27/1 -> SR_Latch7/1
  [VVMC_EstSlope_Deg] -> Switch18/3
  [VTQD_CreepGradeLatch_flg] -> Delay8/1
  Delay4/1 -> Equal51/1
  Equal52/1 -> AND25/2
  SR_Latch7/1 -> [VTQD_CreepGradeLatch_flg]  "VTQD_CreepGradeLatch_flg"
  Constant86/1 -> DelayEnable1/2
  Constant49/1 -> Equal52/2
  Delay5/1 -> Equal53/1
  Constant81/1 -> Equal53/2
  Constant82/1 -> Equal54/2
  Equal53/1 -> AND26/1
  Equal54/1 -> AND26/2
  [VTQD_GearActualPosn_enum] -> Delay5/1
  Abs/1 -> Relational Operator7/1
  Constant85/1 -> Relational Operator7/2
  [VVMC_EstSlope_Deg] -> Abs/1
  Equal51/1 -> AND25/1
  [task_time_s] -> DelayEnable1/3
  Switch18/1 -> [VTQD_CreepCtrlGrade_Deg], Delay9/1  "VTQD_CreepCtrlGrade_Deg"
  Delay9/1 -> Switch18/1
  DelayEnable1/1 -> SR_Latch7/2
  Constant84/1 -> Relational Operator6/2
  Delay8/1 -> DelayEnable1/1
  [VTQD_GearActualPosn_enum] -> Equal54/1
  AND25/1 -> OR18/1
  [VTQD_GearActualPosn_enum] -> Equal52/1
  Constant83/1 -> AND27/2
  Relational Operator7/1 -> AND27/4
  AND26/1 -> OR18/2
  OR18/1 -> AND27/1
  [VTQD_VehActSpd_kph] -> Relational Operator6/1
  Relational Operator6/1 -> AND27/3
  [VTQD_CreepGradeLatch_flg] -> Switch18/2
  [VTQD_GearActualPosn_enum] -> Delay4/1
  [VTQD_VehActSpd_kph] -> MTQD_APSCreepBaseTqD_Z_Nm/2
  [VTQD_CreepCtrlGrade_Deg] -> MTQD_APSCreepBaseTqD_Z_Nm/1
  MTQD_APSCreepBaseTqD_Z_Nm/1 -> [VTQD_APSCreepBaseTqD_Nm]  "VTQD_APSCreepBaseTqD_Nm"
  MTQD_APSCreepBaseTqR_Z_Nm/1 -> [VTQD_APSCreepBaseTqR_Nm]  "VTQD_APSCreepBaseTqR_Nm"
  [VTQD_CreepCtrlGrade_Deg] -> MTQD_APSCreepBaseTqR_Z_Nm/1
  [VTQD_VehActSpd_kph] -> MTQD_APSCreepBaseTqR_Z_Nm/2
  [VTQD_CreepErrSpd_kph] -> MTQD_APSCreepPterm_Z_Nm/2
  [VTQD_VehActSpd_kph] -> MTQD_APSCreepPterm_Z_Nm/1
  MTQD_APSCreepPterm_Z_Nm/1 -> [VTQD_APSCreepPterm_c]  "VTQD_APSCreepPterm_c"
  [VTQD_VehActSpd_kph] -> MTQD_APSCreepIterm_Z_Nm/1
  MTQD_APSCreepIterm_Z_Nm/1 -> [VTQD_APSCreepIterm_c]  "VTQD_APSCreepIterm_c"
  [VTQD_CreepErrSpd_kph] -> MTQD_APSCreepIterm_Z_Nm/2
  [VTQD_CreepBaseTqD_Nm] -> Switch19/3
  [VTQD_APSCreepBaseTqD_Nm] -> Switch19/1
  Switch19/1 -> [VTQD_CreepBaseTqDInp_Nm]  "VTQD_CreepBaseTqDInp_Nm"
  Switch20/1 -> [VTQD_CreepBaseTqRInp_Nm]  "VTQD_CreepBaseTqRInp_Nm"
  [VTQD_APSCreepBaseTqR_Nm] -> Switch20/1
  [VTQD_CreepBaseTqR_Nm] -> Switch20/3
  [VTQD_CreepPterm_c] -> Switch21/3
  [VTQD_APSCreepPterm_c] -> Switch21/1
  Switch21/1 -> [VTQD_CreepPtermInp_c]  "VTQD_CreepPtermInp_c"
  Switch22/1 -> [VTQD_CreepItermInp_c]  "VTQD_CreepItermInp_c"
  [VTQD_APSCreepIterm_c] -> Switch22/1
  [VTQD_CreepIterm_c] -> Switch22/3
  OR19/1 -> Switch19/2
  [VVMC_APSActive_flg] -> OR19/1
  Constant87/1 -> OR19/2
  Constant88/1 -> OR20/2
  [VVMC_APSActive_flg] -> OR20/1
  OR20/1 -> Switch20/2
  Constant89/1 -> OR21/2
  [VVMC_APSActive_flg] -> OR21/1
  OR21/1 -> Switch21/2
  [VVMC_APSActive_flg] -> OR22/1
  Constant90/1 -> OR22/2
  OR22/1 -> Switch22/2
  [VVMC_APSActive_flg] -> If Action Subsystem1/6(VVMC_APSActive_flg)
  [VDDM_EPB1Err_flg] -> Logical Operator8/1
  [VDDM_VehMalfunLevel_enum] -> Equal55/1
  Equal55/1 -> Logical Operator15/1
  Constant94/1 -> Equal55/2
  Constant97/1 -> Logical Operator15/2
  AND5/1 -> OR1/17
  Logical Operator15/1 -> OR1/16
  Constant98/1 -> Logical Operator16/2
  Logical Operator16/1 -> OR23/2
  SR_Latch1/1 -> OR23/1
  Logical Operator10/1 -> Logical Operator16/1
  [VDDM_ESC5Err_flg] -> Logical Operator10/1
  [VTQD_LimpHomeAct_flg] -> Logical Operator9/1
  Constant93/1 -> Switch24/3
  Switch24/1 -> Saturation Dynamic/1  "VTQD_CreepUpLimitTq_Nm"
  Switch14/1 -> Switch24/1
  Constant99/1 -> Logical Operator18/2
  Logical Operator9/1 -> Logical Operator18/1
  Logical Operator18/1 -> Switch24/2
  Switch3/1 -> Switch25/3
  AND29/1 -> Switch25/2
  [VDDM_VCURAPSErrLv2_flg] -> AND29/2
  [VVMC_APSActive_flg] -> AND29/1
  Delay10/1 -> Switch25/1
  Switch25/1 -> Add2/1, Delay10/1  "VTQD_ActCreepBaseTq_Nm"
  BSCPIn_outputs/1 -> Bus Selector/1
  BSignalConvert_outputs/1 -> Bus Selector1/1
  BFunction_outputs/1 -> Bus Selector2/1
  Bus Selector/1 -> [VTQD_LowIdleAccPedal_flg]  "<VTQD_LowIdleAccPedal_flg>"
  Bus Selector2/1 -> [VTQD_GearActualPosn_enum]  "<VTQD_GearActualPosn_enum>"
  Bus Selector/2 -> [VINP_VehSpeed_kph]  "<VINP_VehSpeed_kph>"
  Bus Selector1/1 -> [VTQD_RegenMode_enum]  "<VTQD_RegenMode_enum>"
  Bus Selector/3 -> [VINP_AVHActive_flg]  "<VINP_AVHActive_flg>"
  Bus Selector/4 -> [VTQD_ActBPSPosn_pct]  "<VTQD_ActBPSPosn_pct>"
  Bus Selector/5 -> [VINP_RrRBCActive_flg]  "<VINP_RrRBCActive_flg>"
  Bus Selector/6 -> [VINP_FrEDURealTMTq_Nm]  "<VINP_FrEDURealTMTq_Nm>"
  Bus Selector/7 -> [VINP_RrEDURealTMTq_Nm]  "<VINP_RrEDURealTMTq_Nm>"
  Bus Selector/8 -> [VINP_FrRBCActive_flg]  "<VINP_FrRBCActive_flg>"
  Bus Selector/9 -> [VVMC_ADASActive_flg]  "<VVMC_ADASActive_flg>"
  Bus Selector/10 -> [task_time_s]  "<task_time_s>"
  Bus Selector/11 -> [VVMC_APSSpeedCMD_kph]  "<VVMC_APSSpeedCMD_kph>"
  Bus Selector/12 -> [VVMC_APSActive_flg]  "<VVMC_APSActive_flg>"
  Bus Selector1/2 -> [VTQD_TMRotateDirction_enum]  "<VTQD_TMRotateDirction_enum>"
  Bus Selector1/3 -> [VTQD_RDCActive_enum]  "<VTQD_RDCActive_enum>"
  Bus Selector/13 -> [VVMC_APSReq_enum]  "<VVMC_APSReq_enum>"
  VTQD_PreLoadPreEn_flg/1 -> [VTQD_PreLoadPreEn_flg]
  Bus Selector/14 -> [VVMC_EstSlope_Deg]  "<VVMC_EstSlope_Deg>"
  Bus Selector/15 -> [VPMM_PwrSta_enum]  "<VPMM_PowerSta_enum>"
  Bus Selector/16 -> [VINP_EPBSta_enum]  "<VINP_EPBSta_enum>"
  Bus Selector/17 -> [VTQD_ActAPSPosn_pct]  "<VTQD_ActAPSPosn_pct>"
  Bus Selector/18 -> [VVMC_CAASActive_flg]  "<VVMC_CAASActive_flg>"
  VTQD_PedAccTqEn_flg/1 -> [VTQD_PedAccTqEn_flg]
  Bus Selector/19 -> [VINP_FrPTCSActive_flg]  "<VINP_FrPTCSActive_flg>"
  Bus Selector/20 -> [VINP_RrPTCSActive_flg]  "<VINP_RrPTCSActive_flg>"
  Bus Selector1/4 -> [VTQD_BrkSwSta_flg]  "<VTQD_BrkSwSta_flg>"
  Bus Selector2/2 -> [VTQD_ActWhlSkipSta_enum]  "<VTQD_ActWhlSkipSta_enum>"
  Bus Selector/21 -> [VDDM_EPB1Err_flg]  "<VDDM_EPB1Err_flg>"
  Bus Selector/22 -> [VDDM_ESC5Err_flg]  "<VDDM_ESC5Err_flg>"
  Bus Selector/24 -> [VDDM_VehMalfunLevel_enum]  "<VDDM_VehMalfunLevel_enum>"
  Bus Selector/23 -> [VDDM_EPBSigErrCFS_flg]  "<VDDM_EPBSigErrCFS_flg>"
  Bus Selector/25 -> [VTQD_LimpHomeAct_flg]  "<VTQD_LimpHomeAct_flg>"
  Bus Selector/26 -> [VDDM_VCURAPSErrLv2_flg]  "<VDDM_VCURAPSErrLv2_flg>"
  [VTQD_CreepEnable_flg] -> VTQD_CreepEnable_flg/1
  [VTQD_CreepWhlTqDem_Nm] -> VTQD_CreepWhlTqDem_Nm/1
  [VTQD_CreepPrLoadEnable_flg] -> VTQD_CreepPrLoadEnable_flg/1
  [VTQD_OPDOn2Off_flg] -> VTQD_OPDOn2Off_flg/1
  [VTQD_CreepProtTqEn_flg] -> VTQD_CreepProtTqEn_flg/1
  [VTQD_CreepBaseTqD_Nm] -> VTQD_CreepBaseTqD_Nm/1
  [VTQD_CreepBaseTqR_Nm] -> VTQD_CreepBaseTqR_Nm/1
  [VTQD_HighBPSPosn_flg] -> VTQD_HighBPSPosn_flg/1
  [VTQD_CreepTCSActive_flg] -> VTQD_CreepTCSActive_flg/1
  Bus Selector1/5 -> [VTQD_VehActSpd_kph]  "<VTQD_VehActSpd_kph>"
  Logical Operator/1 -> Data Type Conversion/1
  Relay/1 -> Logical Operator/1
  MTQD_CreepPreloadTime_Y_s/1 -> [VTQD_CreepPreloadSetTime_s]  "VTQD_CreepPreloadSetTime_s"
  [VTQD_CreepPreloadSetTime_s] -> Switch17/3
  NOT26/1 -> OR24/4
  [VTQD_LowSkipDisCreep_flg] -> OR24/5
  [VTQD_CreepDisable_flg] -> OR24/3
  [VTQD_ActBPSPosnInRange_flg] -> OR24/1
  [VTQD_OPDOn2Off_flg] -> OR24/2
  OR24/1 -> [VTQD_CreepPICtrlReset_flg]  "VTQD_CreepPICtrlReset_flg"
  [VTQD_CreepEnable_flg] -> NOT26/1
  [VTQD_CreepPICtrlReset_flg] -> If Action Subsystem1/1(VTQD_CreepPICtrlReset_flg)
  Add2/1 -> [VTQD_CreepBaseAddOfsTq_Nm]
  [VTQD_CreepBaseAddOfsTq_Nm] -> Saturation Dynamic/2  "VTQD_CreepBaseAddOfsTq_Nm"
  Bus Selector2/5 -> [VTQD_OPDHoldEnRel_flg]  "<VTQD_OPDHoldEnRel_flg>"
  Bus Selector2/4 -> [VTQD_APSReqTimer_s]  "<VTQD_APSReqTimer_s>"
  Bus Selector2/3 -> [VTQD_APSReq_enum]  "<VTQD_APSReq_enum>"
  Constant22/1 -> Switch11/3
  Constant3/1 -> OR25/2
  [VVMC_APSActive_flg] -> OR25/1
  OR25/1 -> Switch11/2
  Switch11/1 -> Saturation Dynamic/3
  Constant14/1 -> Switch11/1
  [VTQD_MapCreepUpLimitTq_Nm] -> Switch14/3
  MTQD_CreepUpLimitTq_Y_Nm/1 -> [VTQD_MapCreepUpLimitTq_Nm]  "VTQD_MapCreepUpLimitTq_Nm"
  [VTQD_TqTargetShaftSpd_rpm] -> MTQD_CreepUpLimitTq_Y_Nm/1
  Bus Selector1/6 -> [VTQD_TqTargetShaftSpd_rpm]  "<VTQD_TqTargetShaftSpd_rpm>"
  Bus Selector1/7 -> [VTQD_CreepON_flg]  "<VTQD_CreepON_flg>"
